simulink model "buck_example"  (R2019a)
settings: Solver=ode23t  StartTime=0.0  StopTime=30  MaxStep=2e-4  RelTol=1e-4  EnableMultiTasking=on
model workspace (MAT data in the model file):
  Duty = 0.5
libraries: powerlib x12, simulink x2, powerlib_meascontrol x2, eePwmGenerator x1
Description:
  | Copyright 2008-2019 The MathWorks, Inc.
settings Model: Creator=MathWorks  LastModifiedBy=lizi
settings SolverCC: MaxOrder=4  SolverResetMethod=Robust
settings OptimizationCC: LifeSpan=inf
settings DebuggingCC: ReadBeforeWriteMsg=DisableAll  WriteAfterWriteMsg=DisableAll  WriteAfterReadMsg=DisableAll  MultiTaskDSMMsg=none  SFUnexpectedBacktrackingDiag=warning  SFNoUnconditionalDefaultTransitionDiag=warning  SFExecutionAtInitializationDiag=none  ArithmeticOperatorsInVariantConditions=warning
settings ModelReferenceCC: UpdateModelReferenceTargets=IfOutOfDate
settings SFSimCC: SFSimEcho=off  SimUseLocalCustomCode=off
settings RTWCC: RTWUseLocalCustomCode=off
settings CodeAppCC: StateflowObjectComments=on
settings GRTTargetCC: TargetLangStandard=C89/C90 (ANSI)
settings ConfigComp: CovMetricSettings=dw  CovSaveCumulativeToWorkspaceVar=on  CovSaveSingleToWorkspaceVar=on  CovExternalEMLEnable=off
settings SimscapeCC: SimscapeNormalizeSystem=off  SimscapeNominalValues={1, 'bar'; 1, 'cm^3/s'; 1, 'bar*kg/s'; 1, 'kJ/kg'; 1, 'kW'; }

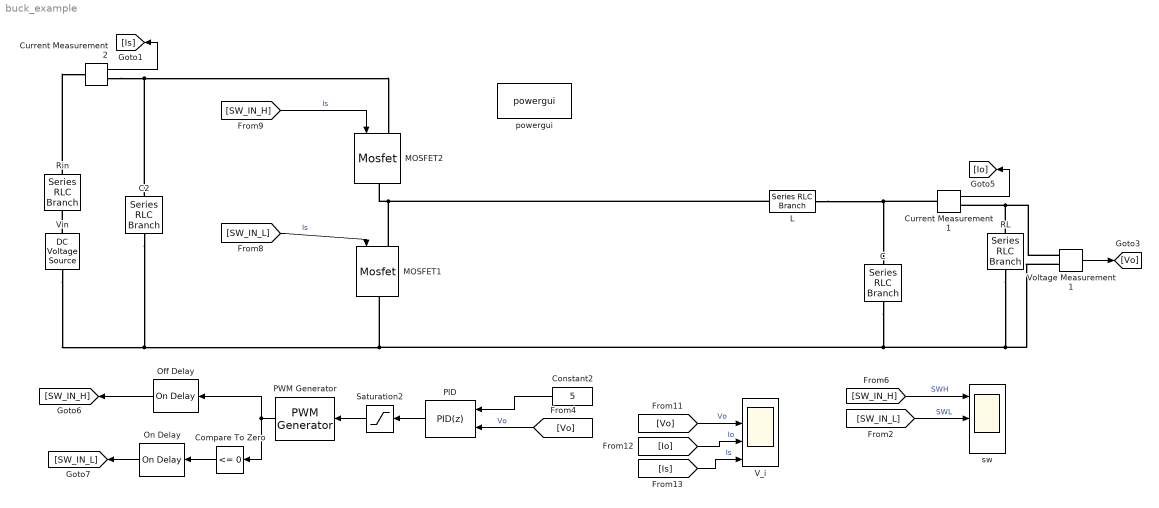
== system buck_example ==
  C : powerlib/Elements/Series RLC Branch  LConnTagsString=__new0  RConnTagsString=__new0  BranchType=RC  Resistance=20e-3  Inductance=200e-6  SetiL0=off  InitialCurrent=0  Capacitance=47e-6  Setx0=off  InitialVoltage=0  Measurements=None
      settings: SourceProductName=Simscape Electrical
  C2 : powerlib/Elements/Series RLC Branch  LConnTagsString=__new0  RConnTagsString=__new0  BranchType=RC  Resistance=20e-3  Inductance=200e-6  SetiL0=off  InitialCurrent=0  Capacitance=100e-6  Setx0=on  InitialVoltage=24  Measurements=None
      settings: SourceProductName=Simscape Electrical
  Compare To Zero : simulink/Logic and Bit Operations/Compare To Zero  relop=<=  OutDataTypeStr=boolean
  Constant2 : Constant  Value=5
  Current Measurement1 : powerlib/Measurements/Current Measurement  PhasorSimulation=off  OutputType=Complex  PSBequivalent=0
      settings: SourceProductName=Simscape Electrical
  Current Measurement2 : powerlib/Measurements/Current Measurement  PhasorSimulation=off  OutputType=Complex  PSBequivalent=0
      settings: SourceProductName=Simscape Electrical
  L : powerlib/Elements/Series RLC Branch  LConnTagsString=__new0  RConnTagsString=__new0  BranchType=RL  Resistance=0.1  Inductance=22e-6  SetiL0=on  InitialCurrent=0  Capacitance=400e-6  Setx0=off  InitialVoltage=0  Measurements=Branch current
      settings: SourceProductName=Simscape Electrical
  MOSFET1 : powerlib/Power Electronics/Mosfet  Ron=10e-3  Lon=0  Rd=1e-3  Vfd=0.6  IC=0  Rs=2  Cs=200e-12  Measurements=off
      settings: SourceProductName=Simscape Electrical
  MOSFET2 : powerlib/Power Electronics/Mosfet  Ron=10e-3  Lon=0  Rd=1e-3  Vfd=0.6  IC=0  Rs=2  Cs=200e-12  Measurements=off
      settings: SourceProductName=Simscape Electrical
  Off Delay : powerlib_meascontrol/Logic/On Delay  DelayType=On delay  delay=50e-9  ic=0  Ts=0
      settings: SourceProductName=Simscape Electrical
  On Delay : powerlib_meascontrol/Logic/On Delay  DelayType=On delay  delay=50e-9  ic=0  Ts=0
      settings: SourceProductName=Simscape Electrical
  PID : simulink/Continuous/PID Controller (2DOF)  Controller=PID  Form=Parallel  TimeDomain=Discrete-time  SampleTime=2e-6  IntegratorMethod=Forward Euler  FilterMethod=Forward Euler  ControllerParametersSource=internal  P=0.084223  I=2051.3241  D=1.6379e-06  UseFilter=on  N=224470.3703  b=1  c=1  TunerSelectOption=Frequency Response Based  InitialConditionSource=internal  InitialConditionForIntegrator=0  InitialConditionForFilter=0  DifferentiatorICPrevScaledInput=0  ExternalReset=none  TrackingMode=off  Kt=1  LimitOutput=off  UpperSaturationLimit=0.9  LowerSaturationLimit=0.01  LinearizeAsGain=off  AntiWindupMode=clamping  Kb=1  POutMin=[]  POutMax=[]  IOutMin=[]  IOutMax=[]  DOutMin=[]  DOutMax=[]  NOutMin=[]  NOutMax=[]  bOutMin=[]  bOutMax=[]  cOutMin=[]  cOutMax=[]  SumOutMin=[]  SumOutMax=[]  SaturationOutMin=[]  SaturationOutMax=[]  PParamMin=[]  PParamMax=[]  IParamMin=[]  IParamMax=[]  DParamMin=[]  DParamMax=[]  NParamMin=[]  NParamMax=[]  bParamMin=[]  bParamMax=[]  cParamMin=[]  cParamMax=[]  KbParamMin=[]  KbParamMax=[]  KtParamMin=[]  KtParamMax=[]  KbOutMin=[]  KbOutMax=[]  KtOutMin=[]  KtOutMax=[]  IntegratorOutMin=[]  IntegratorOutMax=[]  FilterOutMin=[]  FilterOutMax=[]  SumI1OutMin=[]  SumI1OutMax=[]  SumI2OutMin=[]  SumI2OutMax=[]  SumI3OutMin=[]  SumI3OutMax=[]  SumI4OutMin=[]  SumI4OutMax=[]  SumDOutMin=[]  SumDOutMax=[]  Sum1OutMin=[]  Sum1OutMax=[]  Sum2OutMin=[]  Sum2OutMax=[]  Sum3OutMin=[]  Sum3OutMax=[]  DifferentiatorOutMin=[]  DifferentiatorOutMax=[]  FilterDiffOutCoefMin=[]  FilterDiffOutCoefMax=[]  ReciprocalOutMin=[]  ReciprocalOutMax=[]  SumDenOutMin=[]  SumDenOutMax=[]  SumNumOutMin=[]  SumNumOutMax=[]  DivideOutMin=[]  DivideOutMax=[]  IntegratorContinuousStateAttributes=''  IntegratorStateMustResolveToSignalObject=off  IntegratorRTWStateStorageClass=Auto  FilterContinuousStateAttributes=''  FilterStateMustResolveToSignalObject=off  FilterRTWStateStorageClass=Auto  ParallelPVariant=InternalParameters  IdealPVariant=Disabled  IVariant=InternalParameters  DVariant=InternalParameters  bVariant=InternalParameters  cVariant=InternalParameters  IntegratorVariant=Discrete  SatVariant=Disabled  AWVariant=Passthrough  PCopyVariant=Disabled  TRVariant=Disabled  FdbkBlocksVariant=Forward  IdealPFdbkVariant=Disabled  SatFdbkVariant=Disabled  DerivativeFilterVariant=ForwardEulerFilter  NVariant=InternalParameters  NCopyVariant=Disabled  FilterICVariant=InternalICsFilter  IntegratorICVariant=InternalICs  ExternalResetVariant=Disabled  TRSumVariant=Passthrough  SumFdbkVariant=Disabled  SumVariant=Sum_PID
  PWM Generator : eePwmGenerator/PWM Generator  CarrCount=Up  Tper=2e-6  Ts=0
      settings: SourceProductName=Simscape Electrical
  RL : powerlib/Elements/Series RLC Branch  LConnTagsString=__new0  RConnTagsString=__new0  BranchType=R  Resistance=200  Inductance=200e-6  SetiL0=off  InitialCurrent=0  Capacitance=5  Setx0=on  InitialVoltage=0  Measurements=None
      settings: SourceProductName=Simscape Electrical
  Rin : powerlib/Elements/Series RLC Branch  LConnTagsString=__new0  RConnTagsString=__new0  BranchType=R  Resistance=50e-3  Inductance=200e-6  SetiL0=off  InitialCurrent=0  Capacitance=47e-6  Setx0=on  InitialVoltage=24  Measurements=None
      settings: SourceProductName=Simscape Electrical
  Saturation2 : Saturate  UpperLimit=0.95  LowerLimit=0.05
  V_i : Scope  NumInputPorts=4
  Vin : powerlib/Electrical Sources/DC Voltage Source  Amplitude=24  Measurements=None
      settings: SourceProductName=Simscape Electrical
  Voltage Measurement1 : powerlib/Measurements/Voltage Measurement  PhasorSimulation=off  OutputType=Complex  PSBequivalent=0
      settings: SourceProductName=Simscape Electrical
  powergui : powerlib/powergui  Priority=1  SimulationMode=Continuous  SampleTime=50e-6  frequency=60  Iterations=50  frequencyindice=0  Pbase=100e6  ErrMax=1e-4  UnitsV=kV  UnitsW=MW  buscounter=0  FunctionMessages=off  echomessages=off  EnableUseOfTLC=off  CurrentSourceSwitches=off  DisableSnubberDevices=off  DisableRonSwitches=off  DisableVfSwitches=off  DisplayEquations=off  AutomaticDiscreteSolvers=off  SolverType=Tustin/Backward Euler (TBE)  Interpol=off  ExternalGateDelay=off  methode=off  Ts=100  x0status=blocks  SPID=on  SwTol=0  HookPort=off  NonlinearTolerance=0  nMaxIteration=15  ContinueOnMaxIteration=off  RestoreLinks=warning  ResistiveCurrentMeasurement=off  Frange=[0:2:500]  Ylog=off  Xlog=on  ShowGrid=off  save=off  variable=ZData  structure=0  ZoomFFT=off  StartTime=0.0  cycles=1  DisplayStyle=1  fundamental=60  FreqAxis=off  MaxFrequency=1000  frequencyindicesteady=1  RmsSteady=1  display=off
      settings: SourceProductName=Simscape Electrical
  sw : Scope  NumInputPorts=3
  wires:
  PWM Generator/1 -> Compare To Zero/1, Off Delay/1
  Compare To Zero/1 -> On Delay/1
  [SW_IN_H] -> MOSFET2/1  "Is"
  [SW_IN_L] -> MOSFET1/1  "Is"
  [SW_IN_H] -> sw/1  "SWH"
  [SW_IN_L] -> sw/2  "SWL"
  Voltage Measurement1/1 -> [Vo]
  Current Measurement1/1 -> [Io]
  On Delay/1 -> [SW_IN_L]
  Off Delay/1 -> [SW_IN_H]
  [Vo] -> V_i/2  "Vo"
  [Io] -> V_i/3  "Io"
  Saturation2/1 -> PWM Generator/1
  [Is] -> V_i/4  "Is"
  Current Measurement2/1 -> [Is]
  [Vo] -> PID/2  "Vo"
  PID/1 -> Saturation2/1
  Constant2/1 -> PID/1
  connections:
  L/LConn1 -- MOSFET1/LConn1 -- MOSFET2/RConn1
  Vin/LConn1 -- C2/RConn1 -- RL/RConn1 -- Voltage Measurement1/LConn2 -- C/RConn1 -- MOSFET1/RConn1
  Voltage Measurement1/LConn1 -- RL/LConn1 -- Current Measurement1/RConn1
  C2/LConn1 -- Current Measurement2/RConn1 -- MOSFET2/LConn1
  Vin/RConn1 -- Rin/RConn1
  L/RConn1 -- Current Measurement1/LConn1 -- C/LConn1
  Rin/LConn1 -- Current Measurement2/LConn1
